simulink model "gm_simple_blinking_interface"  (R2017a)
settings: Solver=FixedStepAuto  StartTime=0.0  StopTime=10.0  RelTol=1e-3  EnableMultiTasking=on
settings Model: Creator=mini  LastModifiedBy=mini
settings SolverCC: EnableConcurrentExecution=on  ConcurrentTasks=on  PositivePriorityOrder=on
settings OptimizationCC: BlockReduction=off  ConditionallyExecuteInputs=off  PassReuseOutputArgsAs=Individual arguments  MaxStackSize=64
settings DebuggingCC: AlgebraicLoopMsg=error  ParameterTunabilityLossMsg=error
settings HardwareCC: ProdBitPerPointer=32  ProdBitPerSizeT=32  ProdBitPerPtrDiffT=32  ProdLargestAtomicInteger=Long  ProdLargestAtomicFloat=Double  ProdWordSize=32  ProdHWDeviceType=ARM Compatible->ARM Cortex  TargetBitPerPointer=64  TargetBitPerSizeT=64  TargetBitPerPtrDiffT=64  TargetLongLongMode=on  TargetIntDivRoundTo=Zero  TargetEndianess=LittleEndian  TargetWordSize=64  TargetHWDeviceType=MATLAB Host
settings SFSimCC: MATLABDynamicMemAlloc=off
settings RTWCC: SystemTargetFile=ert.tlc  HardwareBoard=ZedBoard  TLCOptions="-aInlineSetEventsForThisBaseRateFcn=TLC_FALSE -aSuppressMultiTaskScheduler=TLC_FALSE  -aRateBasedStepFcn=0"  TemplateMakefile=ert_default_tmf  Description=Embedded Coder  GenerateReport=on  Toolchain=Xilinx Software Development Kit (SDK)  IncludeHyperlinkInReport=on  LaunchReport=on  GenerateTraceInfo=on  GenerateTraceReport=on  GenerateTraceReportSl=on  GenerateTraceReportSf=on  GenerateTraceReportEml=on
settings CodeAppCC: ForceParamTrailComments=on  IgnoreCustomStorageClasses=off  OperatorAnnotations=on  SimulinkDataObjDesc=on  SFDataObjDesc=on  MATLABFcnDesc=on  InsertBlockDesc=on  MATLABSourceComments=on

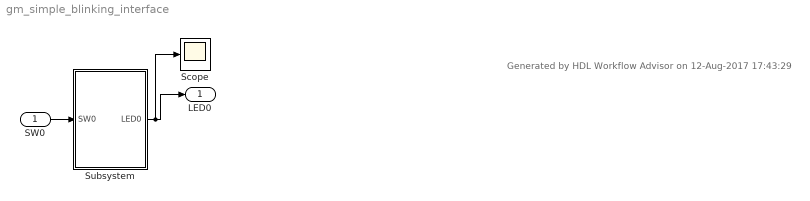
== system gm_simple_blinking_interface ==
  note: Generated by HDL Workflow Advisor on 12-Aug-2017 17:43:29
  SW0 : Inport  OutDataTypeStr=boolean
  Scope : Scope
  Subsystem : Subsystem  TreatAsAtomicUnit=on  mask(AXI4-Lite/AXI4 Interface){}
      mask help:
      | This is an automatically generated subsystem block.
      | This contains the AXI interface blocks that communicate with the simple_bl_ip IPCore generated from simple_blinking/Subsystem subsystem.
      mask Display: disp(sprintf('Xilinx Zynq \nAXI Interface'));
  LED0 : Outport  SampleTime=1
  wires:
  SW0/1 -> Subsystem/1(SW0)
  Subsystem/1(LED0) -> LED0/1, Scope/1

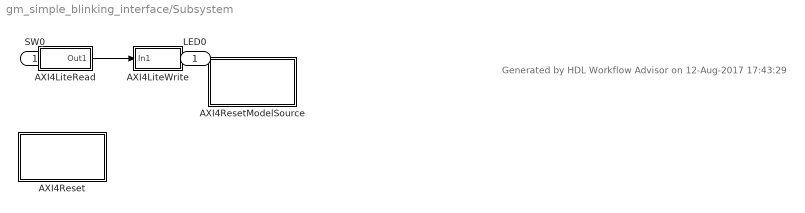
== system gm_simple_blinking_interface/Subsystem ==
  note: Generated by HDL Workflow Advisor on 12-Aug-2017 17:43:29
  SW0 : Inport  OutDataTypeStr=boolean
  AXI4LiteRead : Subsystem  Priority=10
  AXI4LiteWrite : Subsystem  Priority=1
  AXI4Reset : Subsystem  mask(System Start){ShowInLibBrowser=0}
      mask prompts: ShowInLibBrowser "Simulink:masks:CustCodeMaskParam1_MP"
      settings: CopyFcn=cccopyfcn(gcb)  OpenFcn=ccopenfcn('System Start Function')
      mask Help: eval('feval(''rtwprivate'',''rtwhelpview'',''rtw_sys_start_block'')');
      mask Display: disp('System\nStart');
  AXI4ResetModelSource : Subsystem  mask(Model Source){ShowInLibBrowser=0}
      mask prompts: ShowInLibBrowser "Simulink:masks:CustCodeMaskParam1_MP"
      settings: CopyFcn=cccopyfcn(gcb)  OpenFcn=ccopenfcn('Model Source')
      mask Help: eval('feval(''rtwprivate'',''rtwhelpview'',''rtw_model_source_block'')');
      mask Display: disp('Model\nSource');
  LED0 : Outport  SampleTime=1
  wires:
  SW0/1 -> AXI4LiteWrite/1(In1)
  AXI4LiteRead/1(Out1) -> LED0/1

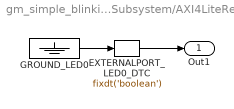
== system gm_simple_blinking_interface/Subsystem/AXI4LiteRead ==
  EXTERNALPORT_LED0_DTC : DataTypeConversion  OutDataTypeStr=fixdt('boolean')
  GROUND_LED0 : Ground
  Out1 : Outport
  wires:
  GROUND_LED0/1 -> EXTERNALPORT_LED0_DTC/1
  EXTERNALPORT_LED0_DTC/1 -> Out1/1

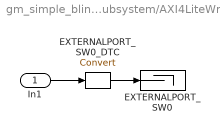
== system gm_simple_blinking_interface/Subsystem/AXI4LiteWrite ==
  In1 : Inport
  EXTERNALPORT_SW0 : Terminator
  EXTERNALPORT_SW0_DTC : DataTypeConversion
  wires:
  In1/1 -> EXTERNALPORT_SW0_DTC/1
  EXTERNALPORT_SW0_DTC/1 -> EXTERNALPORT_SW0/1

== system gm_simple_blinking_interface/Subsystem/AXI4Reset ==

== system gm_simple_blinking_interface/Subsystem/AXI4ResetModelSource ==
